simulink model "test_3ph_core_coupling"  (R2017b)
settings: Solver=VariableStepAuto  StartTime=0.0  StopTime=10.0  RelTol=1e-3
undefined symbols (not defined in the file): Phase, Three
libraries: powerlib x5, typhoonHILlib x1
settings Model: Creator=Marcos  LastModifiedBy=Marcos

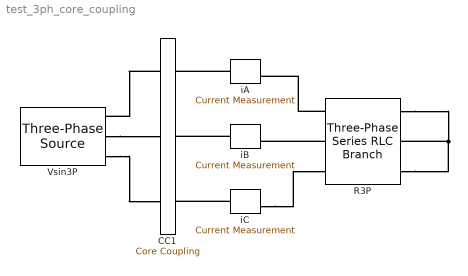
== system test_3ph_core_coupling ==
  CC1 : typhoonHILlib/Core Coupling  CouplingPhases=Three-Phase  IsTLM=off  snb_type_i=None  R1=100e3  C1=1e-6  fixed_snb_i=off  snb_type_v=None  R2=100e3  L1=1e-3  fixed_snb_v=off  CouplingType=Inductive  coup_cap=1e-3  coup_ind=1e-3  toggle_init=on  model_loaded=off  old_pat=typhoonPatterns/TP CC  old_size=15,196
      settings: SourceProductName=Typhoon HIL
  R3P : powerlib/Elements/Three-Phase Series RLC Branch  LConnTagsString=A|B|C  RConnTagsString=A|B|C  BranchType=R  Resistance=10  Inductance=1e-3  Capacitance=1e-6  Measurements=None
  Vsin3P : powerlib/Electrical Sources/Three-Phase Source  InternalConnection=Yn  VoltagePhases=off  Voltage=381  PhaseAngle=0  Voltage_phases=[25e3 25e3 25e3]/sqrt(3)  PhaseAngles_phases=[0 -120 +120]  Frequency=50  NonIdealSource=off  SpecifyImpedance=off  Resistance=0.8929  Inductance=16.58e-3  ShortCircuitLevel=100e6  BaseVoltage=25e3  XRratio=7  BusType=swing  Pref=10e3  Qref=0  Prefabc=[10e3, 10e3, 10e3]  Qrefabc=[0, 0, 0]  Qmin=-inf  Qmax=inf
  iA : powerlib/Measurements/Current Measurement  PhasorSimulation=off  OutputType=Complex  PSBequivalent=0
  iB : powerlib/Measurements/Current Measurement  PhasorSimulation=off  OutputType=Complex  PSBequivalent=0
  iC : powerlib/Measurements/Current Measurement  PhasorSimulation=off  OutputType=Complex  PSBequivalent=0
  connections:
  CC1/LConn1 -- Vsin3P/RConn1
  R3P/LConn1 -- iA/RConn1
  iA/LConn1 -- CC1/RConn1
  Vsin3P/RConn2 -- CC1/LConn2
  R3P/LConn2 -- iB/RConn1
  iC/RConn1 -- R3P/LConn3
  R3P/RConn3 -- R3P/RConn1 -- R3P/RConn2
  iB/LConn1 -- CC1/RConn2
  iC/LConn1 -- CC1/RConn3
  Vsin3P/RConn3 -- CC1/LConn3
